simulink model "Gradient_Identification_Filter"  (R2015b)
settings: Solver=VariableStepAuto  StartTime=0.0  StopTime=10000  FixedStep=1e-3  RelTol=1/36e3
values from neighbouring files (symbols this model uses):
  cell_A123 =     [cells.mat]
  cell_sanyo =     [cells.mat]
undefined symbols (not defined in the file or in its folder): fdesignblkfcn, gcbh
libraries: simulink x2
settings Model: Creator=eprakE  LastModifiedBy=eprakE
settings DebuggingCC: InheritedTsInSrcMsg=none

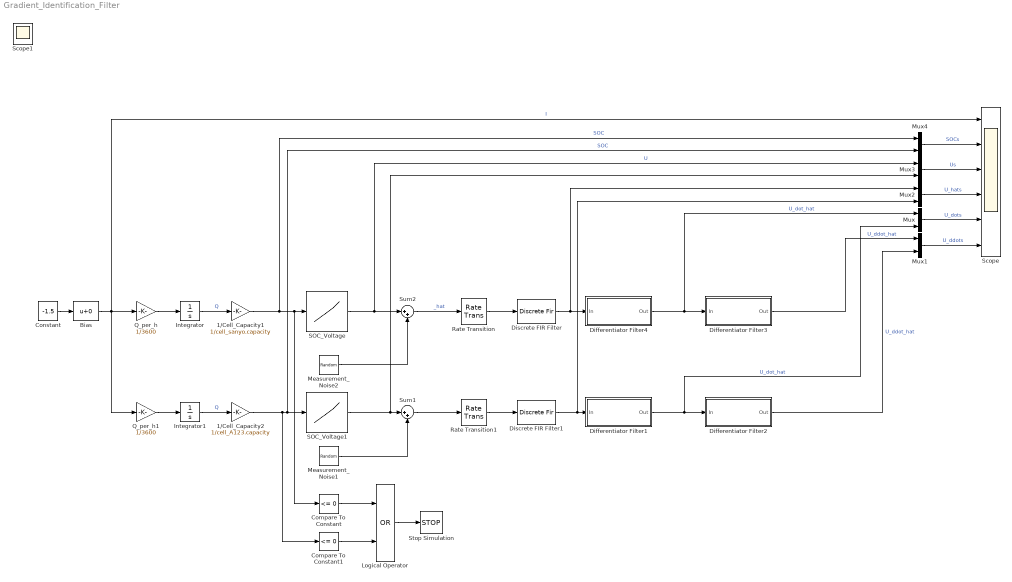
== system Gradient_Identification_Filter ==
  1/Cell_Capacity1 : Gain  Gain=1/cell_sanyo.capacity
  1/Cell_Capacity2 : Gain  Gain=1/cell_A123.capacity
  Bias : Bias
  Compare To Constant : simulink/Logic and Bit Operations/Compare To Constant  relop=<=  const=0  OutDataTypeStr=boolean
  Compare To Constant1 : simulink/Logic and Bit Operations/Compare To Constant  relop=<=  const=0  OutDataTypeStr=boolean
  Constant : Constant  Value=-1.5
  Differentiator Filter1 : Subsystem  DialogController=fdesignblkfcn  InitFcn=fdesignblkfcn(gcbh, {'InitFcn'});  mask(Differentiator Filter){}
      mask help: Design a differentiator filter
      settings: CopyFcn=fdesignblkfcn(gcbh, {'CopyFcn'});
      mask Help: helpview(mapfilelocation('dsp'), 'dspdifferentiatorfilter');
      mask Display: disp('Differentiator');
  Differentiator Filter2 : Subsystem  DialogController=fdesignblkfcn  InitFcn=fdesignblkfcn(gcbh, {'InitFcn'});  mask(Differentiator Filter){}
      mask help: Design a differentiator filter
      settings: CopyFcn=fdesignblkfcn(gcbh, {'CopyFcn'});
      mask Help: helpview(mapfilelocation('dsp'), 'dspdifferentiatorfilter');
      mask Display: disp('Differentiator');
  Differentiator Filter3 : Subsystem  DialogController=fdesignblkfcn  InitFcn=fdesignblkfcn(gcbh, {'InitFcn'});  mask(Differentiator Filter){}
      mask help: Design a differentiator filter
      settings: CopyFcn=fdesignblkfcn(gcbh, {'CopyFcn'});
      mask Help: helpview(mapfilelocation('dsp'), 'dspdifferentiatorfilter');
      mask Display: disp('Differentiator');
  Differentiator Filter4 : Subsystem  DialogController=fdesignblkfcn  InitFcn=fdesignblkfcn(gcbh, {'InitFcn'});  mask(Differentiator Filter){}
      mask help: Design a differentiator filter
      settings: CopyFcn=fdesignblkfcn(gcbh, {'CopyFcn'});
      mask Help: helpview(mapfilelocation('dsp'), 'dspdifferentiatorfilter');
      mask Display: disp('Differentiator');
  Discrete FIR Filter : DiscreteFir  Coefficients=ones(1, 50) * (1/50)
  Discrete FIR Filter1 : DiscreteFir  Coefficients=ones(1, 50) * (1/50)
  Integrator : Integrator  InitialCondition=2
  Integrator1 : Integrator  InitialCondition=1
  Logical Operator : Logic  Operator=OR  AllPortsSameDT=off  OutDataTypeStr=boolean
  Measurement_Noise1 : RandomNumber  Variance=10e-6  Seed=100  SampleTime=1
  Measurement_Noise2 : RandomNumber  Variance=10e-6  SampleTime=1
  Mux{,1..4} (5 alike) : Mux  Inputs=2
  Q_per_h : Gain  Gain=1/3600
  Q_per_h1 : Gain  Gain=1/3600
  Rate Transition : RateTransition  OutPortSampleTime=1
  Rate Transition1 : RateTransition  OutPortSampleTime=1
  SOC_Voltage : Lookup_n-D  NumberOfTableDimensions=1  BreakpointsForDimension1=cell_sanyo.soc  BeginIndexSearchUsingPreviousIndexResult=on  Table=cell_sanyo.voltage  InternalRulePriority=Speed  RndMeth=Simplest  InputSameDT=on
  SOC_Voltage1 : Lookup_n-D  NumberOfTableDimensions=1  BreakpointsForDimension1=cell_A123.soc  BeginIndexSearchUsingPreviousIndexResult=on  Table=cell_A123.voltage  InternalRulePriority=Speed  RndMeth=Simplest  InputSameDT=on
  Scope : Scope  NumInputPorts=6
  Stop Simulation : Stop
  Sum1 : Sum  Inputs=|++
  Sum2 : Sum  Inputs=|++
  Scope1 : Scope
  wires:
  Measurement_Noise2/1 -> Sum2/2
  Integrator/1 -> 1/Cell_Capacity1/1  "Q"
  1/Cell_Capacity1/1 -> Compare To Constant/1, SOC_Voltage/1, Mux4/1  "SOC"
  Constant/1 -> Bias/1
  SOC_Voltage/1 -> Mux3/1, Sum2/1  "U"
  Sum2/1 -> Rate Transition/1  "_hat"
  Bias/1 -> Q_per_h/1, Scope/1, Q_per_h1/1  "I"
  Differentiator Filter4/1(Out) -> Differentiator Filter3/1(In), Mux/1  "U_dot_hat"
  Differentiator Filter3/1(Out) -> Mux1/1  "U_ddot_hat"
  Measurement_Noise1/1 -> Sum1/2
  SOC_Voltage1/1 -> Mux3/2, Sum1/1
  Differentiator Filter1/1(Out) -> Differentiator Filter2/1(In), Mux/2  "U_dot_hat"
  Differentiator Filter2/1(Out) -> Mux1/2  "U_ddot_hat"
  Mux/1 -> Scope/5  "U_dots"
  Mux1/1 -> Scope/6  "U_ddots"
  Integrator1/1 -> 1/Cell_Capacity2/1  "Q"
  1/Cell_Capacity2/1 -> Compare To Constant1/1, Mux4/2, SOC_Voltage1/1  "SOC"
  Logical Operator/1 -> Stop Simulation/1
  Compare To Constant/1 -> Logical Operator/1
  Compare To Constant1/1 -> Logical Operator/2
  Mux2/1 -> Scope/4  "U_hats"
  Sum1/1 -> Rate Transition1/1
  Mux3/1 -> Scope/3  "Us"
  Mux4/1 -> Scope/2  "SOCs"
  Q_per_h/1 -> Integrator/1
  Q_per_h1/1 -> Integrator1/1
  Discrete FIR Filter/1 -> Mux2/1, Differentiator Filter4/1(In)
  Discrete FIR Filter1/1 -> Differentiator Filter1/1(In), Mux2/2
  Rate Transition1/1 -> Discrete FIR Filter1/1
  Rate Transition/1 -> Discrete FIR Filter/1

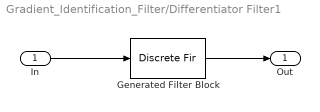
== system Gradient_Identification_Filter/Differentiator Filter1 ==
  In : Inport
  Generated Filter Block : DiscreteFir  Tag=BlockMethodSubSystem  Coefficients=[6.8888672507598612e-06 1.9785794647268016e-05 4.3935018664960248e-05 8.1131672781498989e-05 0.00013029662845138139 0.00018516853568591922 0.00023278751717461436 0.00025318660230508284 0.00022100477798240741 0.00010947407311880585 -0.00010325818300123738 -0.00042612208341097867 -0.00084677364096250084 -0.0013247884382186015 -0.0017885002913050961 -0.0021373749633508514 -0.0022510955637524577 -0.0020053428442092999 -0.0012928034497056221 -4.65142188712242e-05 0.001738457750195441 0.0039894606948889808 0.0065508793446607087 0.0091916874404210543 0.011626653884138085 0.013549453482644705 0.01467351075424724 0.014774547676546949 0.013727909886945146 0.011534072082356968 0.0083273256762509684 0.0043652814461361544 0 -0.0043652814461361544 -0.0083273256762509684 -0.011534072082356968 -0.013727909886945146 -0.014774547676546949 -0.01467351075424724 -0.013549453482644705 -0.011626653884138085 -0.0091916874404210543 -0.0065508793446607087 -0.0039894606948889808 -0.001738457750195441 4.65142188712242e-05 0.0012928034497056221 0.0020053428442092999 0.0022510955637524577 0.0021373749633508514 0.0017885002913050961 0.0013247884382186015 0.00084677364096250084 0.00042612208341097867 0.00010325818300123738 -0.00010947407311880585 -0.00022100477798240741 -0.00025318660230508284 -0.00023278751717461436 -0.00018516853568591922 -0.00013029662845138139 -8.1131672781498989e-05 -4.3935018664960248e-05 -1.9785794647268016e-05 -6.8888672507598612e-06]
  Out : Outport
  wires:
  In/1 -> Generated Filter Block/1
  Generated Filter Block/1 -> Out/1

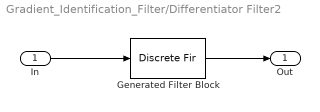
== system Gradient_Identification_Filter/Differentiator Filter2 ==
  In : Inport
  Generated Filter Block : DiscreteFir  Tag=BlockMethodSubSystem  Coefficients=[6.8888672507598612e-06 1.9785794647268016e-05 4.3935018664960248e-05 8.1131672781498989e-05 0.00013029662845138139 0.00018516853568591922 0.00023278751717461436 0.00025318660230508284 0.00022100477798240741 0.00010947407311880585 -0.00010325818300123738 -0.00042612208341097867 -0.00084677364096250084 -0.0013247884382186015 -0.0017885002913050961 -0.0021373749633508514 -0.0022510955637524577 -0.0020053428442092999 -0.0012928034497056221 -4.65142188712242e-05 0.001738457750195441 0.0039894606948889808 0.0065508793446607087 0.0091916874404210543 0.011626653884138085 0.013549453482644705 0.01467351075424724 0.014774547676546949 0.013727909886945146 0.011534072082356968 0.0083273256762509684 0.0043652814461361544 0 -0.0043652814461361544 -0.0083273256762509684 -0.011534072082356968 -0.013727909886945146 -0.014774547676546949 -0.01467351075424724 -0.013549453482644705 -0.011626653884138085 -0.0091916874404210543 -0.0065508793446607087 -0.0039894606948889808 -0.001738457750195441 4.65142188712242e-05 0.0012928034497056221 0.0020053428442092999 0.0022510955637524577 0.0021373749633508514 0.0017885002913050961 0.0013247884382186015 0.00084677364096250084 0.00042612208341097867 0.00010325818300123738 -0.00010947407311880585 -0.00022100477798240741 -0.00025318660230508284 -0.00023278751717461436 -0.00018516853568591922 -0.00013029662845138139 -8.1131672781498989e-05 -4.3935018664960248e-05 -1.9785794647268016e-05 -6.8888672507598612e-06]
  Out : Outport
  wires:
  Generated Filter Block/1 -> Out/1
  In/1 -> Generated Filter Block/1

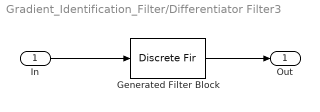
== system Gradient_Identification_Filter/Differentiator Filter3 ==
  In : Inport
  Generated Filter Block : DiscreteFir  Tag=BlockMethodSubSystem  Coefficients=[6.8888672507598612e-06 1.9785794647268016e-05 4.3935018664960248e-05 8.1131672781498989e-05 0.00013029662845138139 0.00018516853568591922 0.00023278751717461436 0.00025318660230508284 0.00022100477798240741 0.00010947407311880585 -0.00010325818300123738 -0.00042612208341097867 -0.00084677364096250084 -0.0013247884382186015 -0.0017885002913050961 -0.0021373749633508514 -0.0022510955637524577 -0.0020053428442092999 -0.0012928034497056221 -4.65142188712242e-05 0.001738457750195441 0.0039894606948889808 0.0065508793446607087 0.0091916874404210543 0.011626653884138085 0.013549453482644705 0.01467351075424724 0.014774547676546949 0.013727909886945146 0.011534072082356968 0.0083273256762509684 0.0043652814461361544 0 -0.0043652814461361544 -0.0083273256762509684 -0.011534072082356968 -0.013727909886945146 -0.014774547676546949 -0.01467351075424724 -0.013549453482644705 -0.011626653884138085 -0.0091916874404210543 -0.0065508793446607087 -0.0039894606948889808 -0.001738457750195441 4.65142188712242e-05 0.0012928034497056221 0.0020053428442092999 0.0022510955637524577 0.0021373749633508514 0.0017885002913050961 0.0013247884382186015 0.00084677364096250084 0.00042612208341097867 0.00010325818300123738 -0.00010947407311880585 -0.00022100477798240741 -0.00025318660230508284 -0.00023278751717461436 -0.00018516853568591922 -0.00013029662845138139 -8.1131672781498989e-05 -4.3935018664960248e-05 -1.9785794647268016e-05 -6.8888672507598612e-06]
  Out : Outport
  wires:
  In/1 -> Generated Filter Block/1
  Generated Filter Block/1 -> Out/1

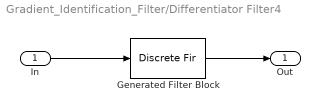
== system Gradient_Identification_Filter/Differentiator Filter4 ==
  In : Inport
  Generated Filter Block : DiscreteFir  Tag=BlockMethodSubSystem  Coefficients=[6.8888672507598612e-06 1.9785794647268016e-05 4.3935018664960248e-05 8.1131672781498989e-05 0.00013029662845138139 0.00018516853568591922 0.00023278751717461436 0.00025318660230508284 0.00022100477798240741 0.00010947407311880585 -0.00010325818300123738 -0.00042612208341097867 -0.00084677364096250084 -0.0013247884382186015 -0.0017885002913050961 -0.0021373749633508514 -0.0022510955637524577 -0.0020053428442092999 -0.0012928034497056221 -4.65142188712242e-05 0.001738457750195441 0.0039894606948889808 0.0065508793446607087 0.0091916874404210543 0.011626653884138085 0.013549453482644705 0.01467351075424724 0.014774547676546949 0.013727909886945146 0.011534072082356968 0.0083273256762509684 0.0043652814461361544 0 -0.0043652814461361544 -0.0083273256762509684 -0.011534072082356968 -0.013727909886945146 -0.014774547676546949 -0.01467351075424724 -0.013549453482644705 -0.011626653884138085 -0.0091916874404210543 -0.0065508793446607087 -0.0039894606948889808 -0.001738457750195441 4.65142188712242e-05 0.0012928034497056221 0.0020053428442092999 0.0022510955637524577 0.0021373749633508514 0.0017885002913050961 0.0013247884382186015 0.00084677364096250084 0.00042612208341097867 0.00010325818300123738 -0.00010947407311880585 -0.00022100477798240741 -0.00025318660230508284 -0.00023278751717461436 -0.00018516853568591922 -0.00013029662845138139 -8.1131672781498989e-05 -4.3935018664960248e-05 -1.9785794647268016e-05 -6.8888672507598612e-06]
  Out : Outport
  wires:
  Generated Filter Block/1 -> Out/1
  In/1 -> Generated Filter Block/1
